simulink model "TPMS"  (R2025a)
settings: Solver=ode4  StartTime=0.0  StopTime=300  FixedStep=0.1  RelTol=1e-3
undefined symbols (not defined in the file): dspblkCoreblockFVToolHelper, gcbh
libraries: simulink x4
settings Model: Creator=Sagar Saini  LastModifiedBy=Sagar Saini

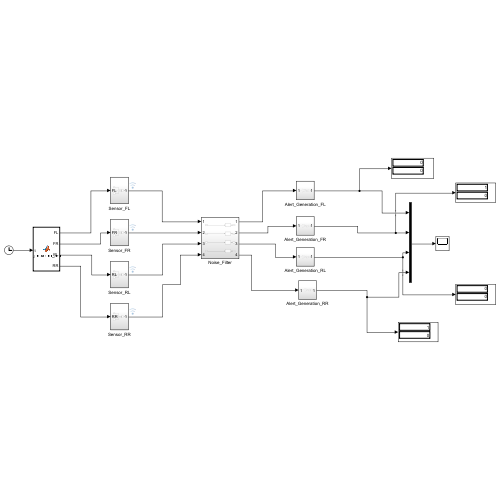
[thumbnail: Simulink's stored preview of the top-level diagram]
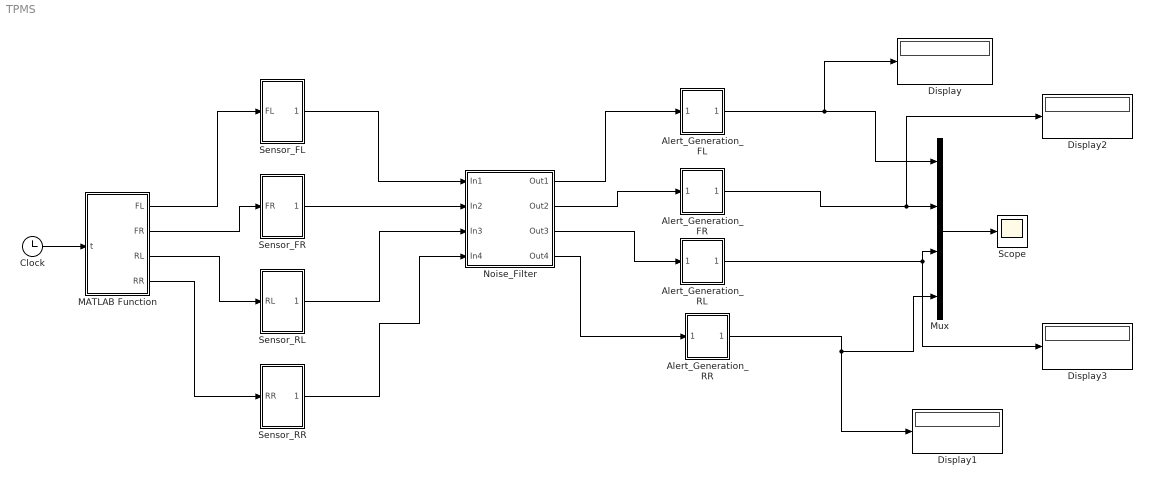
== system TPMS ==
  Alert_Generation_FL : Subsystem
  Alert_Generation_FR : Subsystem
  Alert_Generation_RL : Subsystem
  Alert_Generation_RR : Subsystem
  Clock : Clock
  Display{,1..3} (4 alike) : Display
  MATLAB Function : MATLAB Function  TreatAsAtomicUnit=on
  Mux : Mux
  Noise_Filter : Subsystem
  Scope : Scope
      settings: ActiveDisplayYMinimum=-0.12912890804205523  ActiveDisplayYMaximum=1.1264508990319417
  Sensor_FL : Subsystem
  Sensor_FR : Subsystem
  Sensor_RL : Subsystem
  Sensor_RR : Subsystem
  wires:
  Clock/1 -> MATLAB Function/1(t)
  MATLAB Function/1(FL) -> Sensor_FL/1(FL)
  MATLAB Function/2(FR) -> Sensor_FR/1(FR)
  MATLAB Function/3(RL) -> Sensor_RL/1(RL)
  MATLAB Function/4(RR) -> Sensor_RR/1(RR)
  Sensor_FL/1(Out1) -> Noise_Filter/1(In1)
  Sensor_FR/1(Out1) -> Noise_Filter/2(In2)
  Sensor_RL/1(Out1) -> Noise_Filter/3(In3)
  Sensor_RR/1(Out1) -> Noise_Filter/4(In4)
  Noise_Filter/1(Out1) -> Alert_Generation_FL/1(In1)
  Noise_Filter/2(Out2) -> Alert_Generation_FR/1(In1)
  Noise_Filter/3(Out3) -> Alert_Generation_RL/1(In1)
  Noise_Filter/4(Out4) -> Alert_Generation_RR/1(In1)
  Alert_Generation_FL/1(Out1) -> Display/1, Mux/1
  Alert_Generation_FR/1(Out1) -> Display2/1, Mux/2
  Alert_Generation_RL/1(Out1) -> Mux/3, Display3/1
  Alert_Generation_RR/1(Out1) -> Display1/1, Mux/4
  Mux/1 -> Scope/1

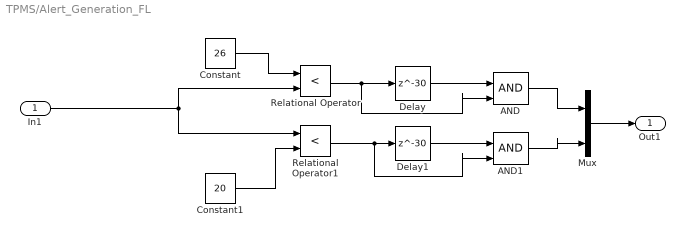
== system TPMS/Alert_Generation_FL ==
  In1 : Inport
  AND : Logic  IconShape=distinctive  AllPortsSameDT=off  OutDataTypeStr=boolean
  AND1 : Logic  IconShape=distinctive  AllPortsSameDT=off  OutDataTypeStr=boolean
  Constant : Constant  Value=26
  Constant1 : Constant  Value=20
  Delay : Delay  DelayLength=30
  Delay1 : Delay  DelayLength=30
  Mux : Mux  Inputs=2
  Relational Operator : RelationalOperator  Operator=<  OutDataTypeStr=boolean  RndMeth=Simplest  InputSameDT=off
  Relational Operator1 : RelationalOperator  Operator=<  OutDataTypeStr=boolean  RndMeth=Simplest  InputSameDT=off
  Out1 : Outport
  wires:
  Relational Operator/1 -> AND/2, Delay/1
  In1/1 -> Relational Operator1/1, Relational Operator/2
  AND/1 -> Mux/1
  Constant/1 -> Relational Operator/1
  Relational Operator1/1 -> AND1/2, Delay1/1
  Constant1/1 -> Relational Operator1/2
  Delay1/1 -> AND1/1
  Delay/1 -> AND/1
  AND1/1 -> Mux/2
  Mux/1 -> Out1/1

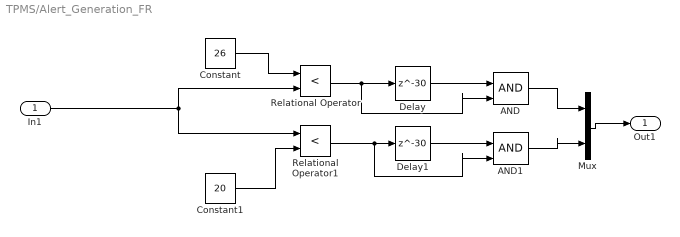
== system TPMS/Alert_Generation_FR ==
  In1 : Inport
  AND : Logic  IconShape=distinctive  AllPortsSameDT=off  OutDataTypeStr=boolean
  AND1 : Logic  IconShape=distinctive  AllPortsSameDT=off  OutDataTypeStr=boolean
  Constant : Constant  Value=26
  Constant1 : Constant  Value=20
  Delay : Delay  DelayLength=30
  Delay1 : Delay  DelayLength=30
  Mux : Mux  Inputs=2
  Relational Operator : RelationalOperator  Operator=<  OutDataTypeStr=boolean  RndMeth=Simplest  InputSameDT=off
  Relational Operator1 : RelationalOperator  Operator=<  OutDataTypeStr=boolean  RndMeth=Simplest  InputSameDT=off
  Out1 : Outport
  wires:
  Mux/1 -> Out1/1
  AND1/1 -> Mux/2
  Delay/1 -> AND/1
  Delay1/1 -> AND1/1
  Constant1/1 -> Relational Operator1/2
  Relational Operator1/1 -> Delay1/1, AND1/2
  Constant/1 -> Relational Operator/1
  AND/1 -> Mux/1
  In1/1 -> Relational Operator/2, Relational Operator1/1
  Relational Operator/1 -> Delay/1, AND/2

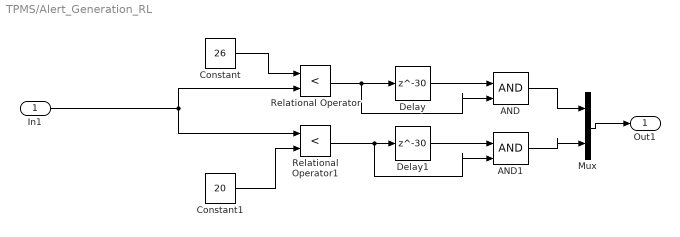
== system TPMS/Alert_Generation_RL ==
  In1 : Inport
  AND : Logic  IconShape=distinctive  AllPortsSameDT=off  OutDataTypeStr=boolean
  AND1 : Logic  IconShape=distinctive  AllPortsSameDT=off  OutDataTypeStr=boolean
  Constant : Constant  Value=26
  Constant1 : Constant  Value=20
  Delay : Delay  DelayLength=30
  Delay1 : Delay  DelayLength=30
  Mux : Mux  Inputs=2
  Relational Operator : RelationalOperator  Operator=<  OutDataTypeStr=boolean  RndMeth=Simplest  InputSameDT=off
  Relational Operator1 : RelationalOperator  Operator=<  OutDataTypeStr=boolean  RndMeth=Simplest  InputSameDT=off
  Out1 : Outport
  wires:
  Relational Operator/1 -> AND/2, Delay/1
  In1/1 -> Relational Operator1/1, Relational Operator/2
  AND/1 -> Mux/1
  Constant/1 -> Relational Operator/1
  Relational Operator1/1 -> AND1/2, Delay1/1
  Constant1/1 -> Relational Operator1/2
  Delay1/1 -> AND1/1
  Delay/1 -> AND/1
  AND1/1 -> Mux/2
  Mux/1 -> Out1/1

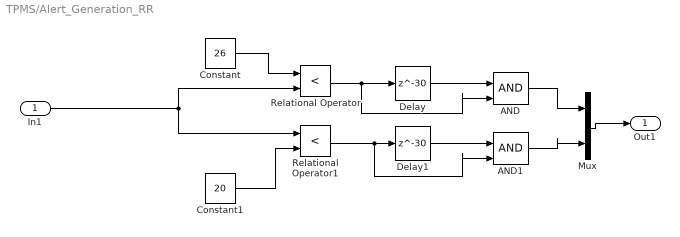
== system TPMS/Alert_Generation_RR ==
  In1 : Inport
  AND : Logic  IconShape=distinctive  AllPortsSameDT=off  OutDataTypeStr=boolean
  AND1 : Logic  IconShape=distinctive  AllPortsSameDT=off  OutDataTypeStr=boolean
  Constant : Constant  Value=26
  Constant1 : Constant  Value=20
  Delay : Delay  DelayLength=30
  Delay1 : Delay  DelayLength=30
  Mux : Mux  Inputs=2
  Relational Operator : RelationalOperator  Operator=<  OutDataTypeStr=boolean  RndMeth=Simplest  InputSameDT=off
  Relational Operator1 : RelationalOperator  Operator=<  OutDataTypeStr=boolean  RndMeth=Simplest  InputSameDT=off
  Out1 : Outport
  wires:
  Mux/1 -> Out1/1
  AND1/1 -> Mux/2
  Delay/1 -> AND/1
  Delay1/1 -> AND1/1
  Constant1/1 -> Relational Operator1/2
  Relational Operator1/1 -> Delay1/1, AND1/2
  Constant/1 -> Relational Operator/1
  AND/1 -> Mux/1
  In1/1 -> Relational Operator/2, Relational Operator1/1
  Relational Operator/1 -> Delay/1, AND/2

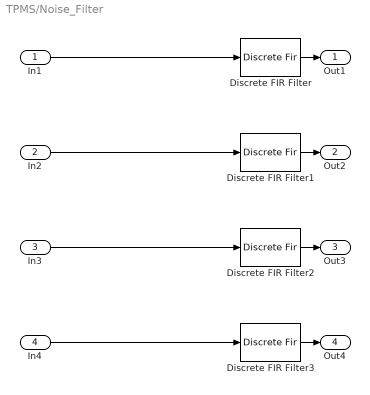
== system TPMS/Noise_Filter ==
  In1 : Inport
  In2 : Inport  Port=2
  In3 : Inport  Port=3
  In4 : Inport  Port=4
  Discrete FIR Filter{,1..3} (4 alike) : DiscreteFir  LoadFcn=dspblkCoreblockFVToolHelper(gcbh,'load');  Coefficients=ones(1,30)/30
      settings: CopyFcn=dspblkCoreblockFVToolHelper(gcbh,'copy');  DeleteFcn=dspblkCoreblockFVToolHelper(gcbh,'close');  ModelCloseFcn=dspblkCoreblockFVToolHelper(gcbh,'close');  PreSaveFcn=dspblkCoreblockFVToolHelper(gcbh,'presave');  PostSaveFcn=dspblkCoreblockFVToolHelper(gcbh,'postsave');  CloseFcn=dspblkCoreblockFVToolHelper(gcbh,'close');
  Out1 : Outport
  Out2 : Outport  Port=2
  Out3 : Outport  Port=3
  Out4 : Outport  Port=4
  wires:
  In1/1 -> Discrete FIR Filter/1
  Discrete FIR Filter/1 -> Out1/1
  In3/1 -> Discrete FIR Filter2/1
  Discrete FIR Filter2/1 -> Out3/1
  In4/1 -> Discrete FIR Filter3/1
  In2/1 -> Discrete FIR Filter1/1
  Discrete FIR Filter3/1 -> Out4/1
  Discrete FIR Filter1/1 -> Out2/1

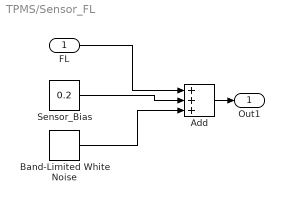
== system TPMS/Sensor_FL ==
  FL : Inport
  Add : Sum  Inputs=+++
  Band-Limited White Noise : simulink/Sources/Band-Limited White Noise  Cov=[0.09]  Ts=0.1  seed=[23341]
  Sensor_Bias : Constant  Value=0.2
  Out1 : Outport
  wires:
  Band-Limited White Noise/1 -> Add/3
  Sensor_Bias/1 -> Add/2
  FL/1 -> Add/1
  Add/1 -> Out1/1

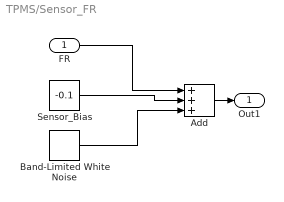
== system TPMS/Sensor_FR ==
  FR : Inport
  Add : Sum  Inputs=+++
  Band-Limited White Noise : simulink/Sources/Band-Limited White Noise  Cov=[0.09]  Ts=0.1  seed=[23341]
  Sensor_Bias : Constant  Value=-0.1
  Out1 : Outport
  wires:
  Add/1 -> Out1/1
  FR/1 -> Add/1
  Sensor_Bias/1 -> Add/2
  Band-Limited White Noise/1 -> Add/3

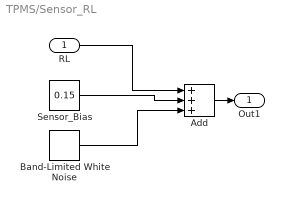
== system TPMS/Sensor_RL ==
  RL : Inport
  Add : Sum  Inputs=+++
  Band-Limited White Noise : simulink/Sources/Band-Limited White Noise  Cov=[0.09]  Ts=0.1  seed=[23341]
  Sensor_Bias : Constant  Value=0.15
  Out1 : Outport
  wires:
  Band-Limited White Noise/1 -> Add/3
  Sensor_Bias/1 -> Add/2
  RL/1 -> Add/1
  Add/1 -> Out1/1

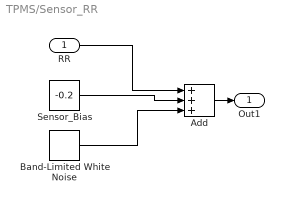
== system TPMS/Sensor_RR ==
  RR : Inport
  Add : Sum  Inputs=+++
  Band-Limited White Noise : simulink/Sources/Band-Limited White Noise  Cov=[0.09]  Ts=0.1  seed=[23341]
  Sensor_Bias : Constant  Value=-0.2
  Out1 : Outport
  wires:
  Add/1 -> Out1/1
  RR/1 -> Add/1
  Sensor_Bias/1 -> Add/2
  Band-Limited White Noise/1 -> Add/3

== matlab function TPMS/MATLAB Function ==
  data: t input; FL output double; FR output double; RL output double; RR output double
function [FL, FR, RL, RR] = tire_pressure_profile(t)
%  Driving phases:
%    Phase 1 :   0 – 60 s  → Highway   (thermal rise)
%    Phase 2 :  60 – 180 s → Urban     (FL slow leak)
%    Phase 3 : 180 – 300 s → Mountain  (RL pothole at t = 200 s)

P_nom = 32.0;   % nominal pressure (PSI)

%% ── PHASE 1 : Highway (0 – 60 s) ─────────────────────────
% Tyres heat up → pressure rises linearly by 0.5 PSI
if t < 60
    thermal = 0.5 * (t / 60);     
    FL = P_nom + thermal;
    FR = P_nom + thermal;
    RL = P_nom + thermal;
    RR = P_nom + thermal;

%% ── PHASE 2 : Urban stop-and-go (60 – 180 s) ────────────
% FL tire has a slow puncture: loses 8 PSI over 120 s
elseif t < 180
    phase_t = t - 60;               
    thermal  = 0.5;                 

    leak_FL = -8.0 * (phase_t / 120);   

    FL = P_nom + thermal + leak_FL;     
    FR = P_nom + thermal;               
    RL = P_nom + thermal;               
    RR = P_nom + thermal;               

%% ── PHASE 3 : Mountain road (180 – 300 s) ───────────────
% FL continues leaking. RL hits a pothole at t = 200 s → rapid deflation.
else
    phase_t = t - 180;              
    thermal  = 0.5 - 0.3 * (phase_t / 120);  


    leak_FL = -8.0 - 4.0 * (phase_t / 120);


    if t < 200
        leak_RL = 0;
    else
        deflate_t = min(t - 200, 30);         
        leak_RL = -12.0 * (deflate_t / 30);  
    end

    FL = max(P_nom + thermal + leak_FL, 0);  
    FR = P_nom + thermal;
    RL = max(P_nom + thermal + leak_RL, 0);   
    RR = P_nom + thermal;
end
